simulink model "HW02_Q2_Thompson"  (R2022a)
settings: Solver=VariableStepAuto  StartTime=0.0  StopTime=10  RelTol=1e-3
values from neighbouring files (symbols this model uses):
  C = 0.00001    (= 1e-05)    [HW1_Q4.m]    (also in Homework01.m = 0.01; Homework1.m = 4.7e-05; ParallelRLC.m = 0.1)
  L = 10    [HW1_Q4.m]    (also in Homework01.m = 5; Homework1.m; ParallelRLC.m = 5)
  R = 100    [HW1_Q4.m]    (also in Homework01.m; Homework1.m; ParallelRLC.m = 5)
settings Model: Creator=kylet  LastModifiedBy=kylet

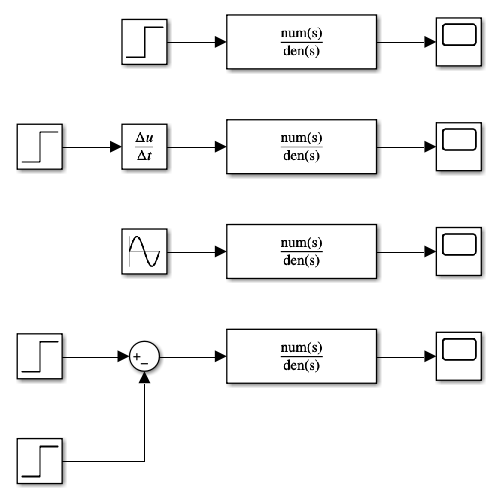
[thumbnail: Simulink's stored preview of the top-level diagram]
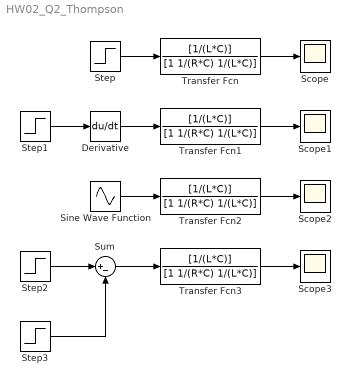
== system HW02_Q2_Thompson ==
  Derivative : Derivative
  Scope{,1..3} (4 alike) : Scope
  Sine Wave Function : Sin  SampleTime=0
  Step : Step  Time=0.01  SampleTime=0
  Step1 : Step  Time=0.01  SampleTime=0
  Step2 : Step  Time=0.01  SampleTime=0
  Step3 : Step  Time=2  SampleTime=0
  Sum : Sum  Inputs=|+-
  Transfer Fcn{,1..3} (4 alike) : TransferFcn  Numerator=[1/(L*C)]  Denominator=[1 1/(R*C) 1/(L*C)]
  wires:
  Step/1 -> Transfer Fcn/1
  Transfer Fcn/1 -> Scope/1
  Transfer Fcn1/1 -> Scope1/1
  Derivative/1 -> Transfer Fcn1/1
  Step1/1 -> Derivative/1
  Transfer Fcn2/1 -> Scope2/1
  Sine Wave Function/1 -> Transfer Fcn2/1
  Step2/1 -> Sum/1
  Step3/1 -> Sum/2
  Transfer Fcn3/1 -> Scope3/1
  Sum/1 -> Transfer Fcn3/1
